simulink model "projectQseven"  (R2023b)
settings: Solver=VariableStepAuto  StartTime=0.0  StopTime=10.0  RelTol=1e-3
libraries: simulink x1
settings Model: Creator=Windows 10 2A-2017  LastModifiedBy=Asus
settings OptimizationCC: ReuseModelBlockBuffer=off

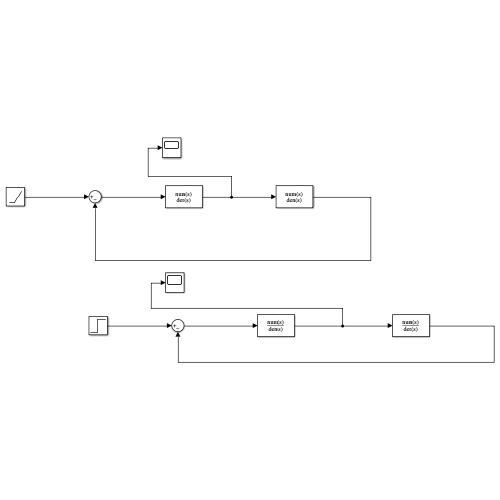
[thumbnail: Simulink's stored preview of the top-level diagram]
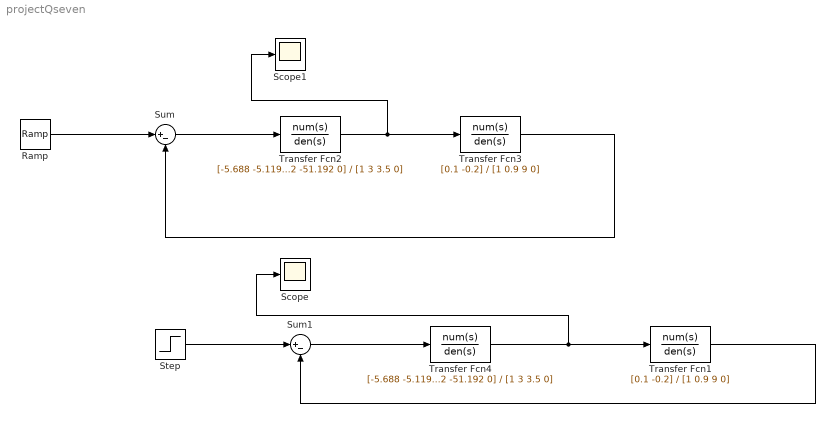
== system projectQseven ==
  Ramp : simulink/Sources/Ramp  slope=1  start=0  InitialOutput=0
  Scope : Scope
  Scope1 : Scope
  Step : Step  SampleTime=0
  Sum : Sum  Inputs=|+-
  Sum1 : Sum  Inputs=|+-
  Transfer Fcn1 : TransferFcn  Numerator=[0.1 -0.2]  Denominator=[1 0.9 9 0]
  Transfer Fcn2 : TransferFcn  Numerator=[-5.688 -5.1192 -51.192 0]  Denominator=[1 3 3.5 0]
  Transfer Fcn3 : TransferFcn  Numerator=[0.1 -0.2]  Denominator=[1 0.9 9 0]
  Transfer Fcn4 : TransferFcn  Numerator=[-5.688 -5.1192 -51.192 0]  Denominator=[1 3 3.5 0]
  wires:
  Transfer Fcn1/1 -> Sum1/2
  Sum1/1 -> Transfer Fcn4/1
  Sum/1 -> Transfer Fcn2/1
  Ramp/1 -> Sum/1
  Transfer Fcn3/1 -> Sum/2
  Step/1 -> Sum1/1
  Transfer Fcn2/1 -> Scope1/1, Transfer Fcn3/1
  Transfer Fcn4/1 -> Scope/1, Transfer Fcn1/1
